simulink model "test_without_actuator"  (R2022b)
settings: Solver=FixedStepAuto  StartTime=0.0  StopTime=10  FixedStep=0.1  RelTol=1e-3
values from neighbouring files (symbols this model uses):
  C_M = 1.1366    [init.m]
  C_T = 3.5611    [init.m]
  D_p = 0.1    [init.m]
  model_param = struct(     'I', I,      'mass', ModelParam_m,      'g', ModelParam_g,      'c_T', ModelParam_c_T,      'c_M', ModelParam_c_M,      'd', ModelParam_d,      'J_RP', ModelParam_J_RP,      'init_pos', [ModelInit_Pos_x, ModelInit_Pos_y, ModelInit_Pos_z],      'init_att', [ModelInit_Att_x, ModelInit_Att_y, ModelInit_Att_z],      'C_T', C_T,      'C_M', C_M,      'air_density', p,      'prop_diameter',  ...(+52 chars)    [init.m]
  ModelInit_Att_qw = 0    [init.m]
  ModelInit_Att_qx = 1    [init.m]
  ModelInit_Att_qy = 0    [init.m]
  ModelInit_Att_qz = 0    [init.m]
  ModelInit_Pos_x = 0    [init.m]
  ModelInit_Pos_y = 0    [init.m]
  ModelInit_Pos_z = 0    [init.m]
  ModelParam_c_M = 1.779e-07*2    (= 3.558e-07)    [init.m]
  ModelParam_c_T = 1.105e-05    [init.m]
  ModelParam_d = 0.225    [init.m]
  ModelParam_g = 9.8    [init.m]
  ModelParam_I_xx = 0.0211    [init.m]
  ModelParam_I_yy = 0.0219    [init.m]
  ModelParam_I_zz = 0.0366    [init.m]
  ModelParam_J_RP = 0.0001287    [init.m]
  ModelParam_m = 1.4    [init.m]
  p = pos(idx,:)    [draw_morecool.m]    (also in init.m = 1.225)
(part 1 of 2)
settings Model: Creator=12854  LastModifiedBy=12854

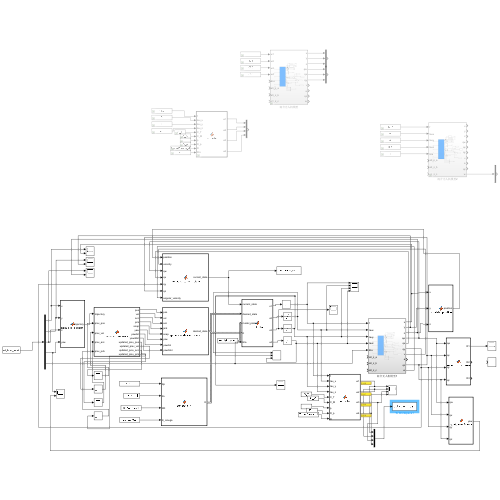
[thumbnail: Simulink's stored preview of the top-level diagram]
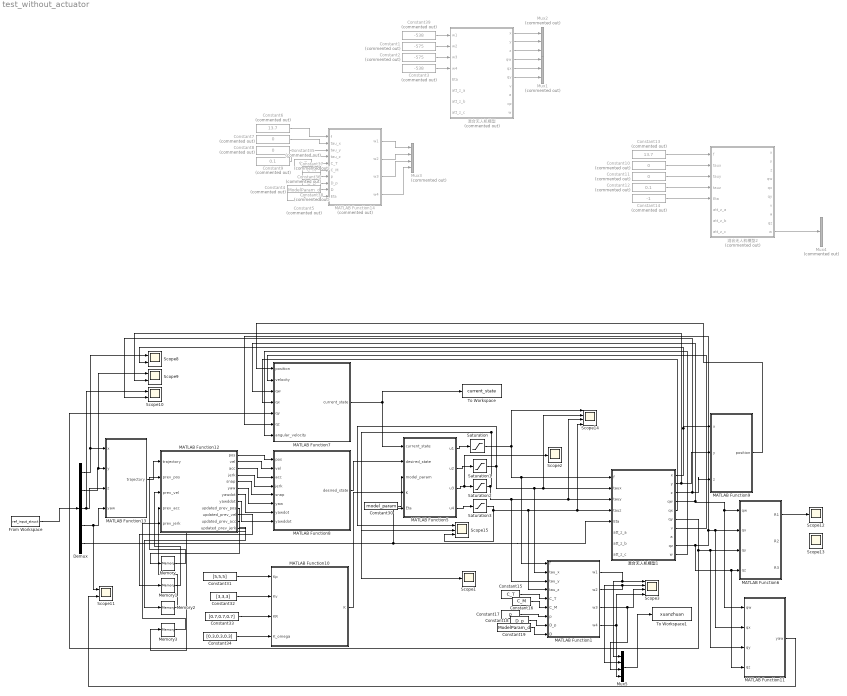
== system test_without_actuator ==
  Constant1 : Constant  Commented=on  Value=-575  SampleTime=0.1
  Constant10 : Constant  Commented=on  Value=0  SampleTime=0.1
  Constant11 : Constant  Commented=on  Value=0  SampleTime=0
  Constant12 : Constant  Commented=on  Value=0.1  SampleTime=0.1
  Constant13 : Constant  Commented=on  Value=13.7  SampleTime=0.1
  Constant14 : Constant  Commented=on  Value=-1  SampleTime=0.1
  Constant15 : Constant  Value=C_T  SampleTime=0.1
  Constant16 : Constant  Value=C_M  SampleTime=0.1
  Constant17 : Constant  Value=p  SampleTime=0.1
  Constant18 : Constant  Value=D_p  SampleTime=0.1
  Constant19 : Constant  Value=ModelParam_d  SampleTime=0.1
  Constant2 : Constant  Commented=on  Value=-575  SampleTime=0.1
  Constant3 : Constant  Commented=on  Value=-538  SampleTime=0.1
  Constant30 : Constant  Value=model_param  OutDataTypeStr=Bus: model_param_bus  SampleTime=0.1
  Constant31 : Constant  Value=[5,5,5]  SampleTime=0.1
  Constant32 : Constant  Value=[3,3,3]  SampleTime=0.1
  Constant33 : Constant  Value=[0.7,0.7,0.7]  SampleTime=0.1
  Constant34 : Constant  Value=[0.3,0.3,0.3]  SampleTime=0.1
  Constant35 : Constant  Commented=on  Value=C_T  SampleTime=0.1
  Constant36 : Constant  Commented=on  Value=C_M  SampleTime=0.1
  Constant37 : Constant  Commented=on  Value=p  SampleTime=0.1
  Constant38 : Constant  Commented=on  Value=D_p  SampleTime=0.1
  Constant39 : Constant  Commented=on  Value=-538  SampleTime=0.1
  Constant4 : Constant  Commented=on  Value=ModelParam_d  SampleTime=0.1
  Constant5 : Constant  Commented=on  Value=-1  SampleTime=0.1
  Constant6 : Constant  Commented=on  Value=13.7  SampleTime=0.1
  Constant7 : Constant  Commented=on  Value=0  SampleTime=0
  Constant8 : Constant  Commented=on  Value=0  SampleTime=0.1
  Constant9 : Constant  Commented=on  Value=0.1  SampleTime=0.1
  Demux : Demux  Outputs=5
  From Workspace : FromWorkspace  VariableName=ref_input_struct  SampleTime=0.1
  MATLAB Function1 : MATLAB Function  TreatAsAtomicUnit=on  SystemSampleTime=0.1
  MATLAB Function10 : MATLAB Function  TreatAsAtomicUnit=on
  MATLAB Function11 : MATLAB Function  TreatAsAtomicUnit=on
  MATLAB Function12 : MATLAB Function  TreatAsAtomicUnit=on
  MATLAB Function13 : MATLAB Function  TreatAsAtomicUnit=on
  MATLAB Function14 : MATLAB Function  Commented=on  TreatAsAtomicUnit=on  SystemSampleTime=0.1
  MATLAB Function5 : MATLAB Function  TreatAsAtomicUnit=on
  MATLAB Function6 : MATLAB Function  TreatAsAtomicUnit=on
  MATLAB Function7 : MATLAB Function  TreatAsAtomicUnit=on  SystemSampleTime=0.1
  MATLAB Function8 : MATLAB Function  TreatAsAtomicUnit=on
  MATLAB Function9 : MATLAB Function  TreatAsAtomicUnit=on
  Memory{,1..3} (4 alike) : Memory  InheritSampleTime=on
  Mux1 : Mux  Commented=on  Inputs=3
  Mux2 : Mux  Commented=on  Inputs=3
  Mux3 : Mux  Commented=on
  Mux4 : Mux  Commented=on  Inputs=1
  Mux5 : Mux
  Saturation : Saturate  UpperLimit=20  LowerLimit=-20
  Saturation1 : Saturate  UpperLimit=0.3  LowerLimit=-0.3
  Saturation2 : Saturate  UpperLimit=0.3  LowerLimit=-0.3
  Saturation3 : Saturate  UpperLimit=0.3  LowerLimit=-0.3
  Scope{1..2,12..13} (4 alike) : Scope
  Scope{8..11} (4 alike) : Scope  NumInputPorts=2
  Scope14 : Scope  NumInputPorts=4
  Scope15 : Scope  NumInputPorts=3
  Scope3 : Scope  NumInputPorts=4
  To Workspace : ToWorkspace  VariableName=current_state  SaveFormat=Timeseries  SampleTime=-1
  To Workspace1 : ToWorkspace  VariableName=xuanzhuan  SaveFormat=Timeseries  SampleTime=-1
  混合无人机模型 : Subsystem  Commented=on
  混合无人机模型1 : Subsystem
  混合无人机模型2 : Subsystem  Commented=on
  wires:
  Constant39/1 -> 混合无人机模型/1(w1)
  Constant1/1 -> 混合无人机模型/2(w2)
  Constant2/1 -> 混合无人机模型/3(w3)
  Constant3/1 -> 混合无人机模型/4(w4)
  混合无人机模型/1(x) -> Mux2/1
  混合无人机模型/2(y) -> Mux2/2
  混合无人机模型/3(z) -> Mux2/3
  混合无人机模型/4(qw) -> Mux1/1
  混合无人机模型/5(qx) -> Mux1/2
  混合无人机模型/6(qy) -> Mux1/3
  Constant35/1 -> MATLAB Function14/5(C_T)
  Constant36/1 -> MATLAB Function14/6(C_M)
  Constant37/1 -> MATLAB Function14/7(p)
  Constant38/1 -> MATLAB Function14/8(D_p)
  Constant4/1 -> MATLAB Function14/9(D)
  Constant5/1 -> MATLAB Function14/10(Eta)
  Constant6/1 -> MATLAB Function14/1(f)
  Constant7/1 -> MATLAB Function14/2(tau_x)
  Constant8/1 -> MATLAB Function14/3(tau_y)
  Constant9/1 -> MATLAB Function14/4(tau_z)
  MATLAB Function14/1(w1) -> Mux3/1
  MATLAB Function14/2(w2) -> Mux3/2
  MATLAB Function14/3(w3) -> Mux3/3
  MATLAB Function14/4(w4) -> Mux3/4
  MATLAB Function13/1(trajectory) -> MATLAB Function12/1(trajectory)
  MATLAB Function12/7(yawdot) -> MATLAB Function8/7(yawdot)
  MATLAB Function10/1(K) -> MATLAB Function5/4(K)
  MATLAB Function5/1(u1) -> Saturation/1
  Demux/1 -> Scope8/1, MATLAB Function13/1(x)
  Demux/2 -> Scope9/1, MATLAB Function13/2(y)
  混合无人机模型1/2(y) -> Scope9/2, MATLAB Function9/2(y)
  MATLAB Function5/4(u4) -> Saturation3/1
  From Workspace/1 -> Demux/1
  混合无人机模型1/7(v) -> MATLAB Function7/2(velocity)
  MATLAB Function6/1(R1) -> Scope12/1
  Constant31/1 -> MATLAB Function10/1(Kp)
  MATLAB Function12/10(updated_prev_vel) -> Memory1/1
  MATLAB Function7/1(current_state) -> MATLAB Function5/1(current_state), To Workspace/1
  混合无人机模型1/3(z) -> Scope10/2, MATLAB Function9/3(z)
  Memory1/1 -> MATLAB Function12/3(prev_vel)
  Constant32/1 -> MATLAB Function10/2(Kv)
  混合无人机模型1/10(w) -> MATLAB Function7/7(angular_velocity)
  Demux/4 -> Scope11/1, MATLAB Function13/4(yaw)
  MATLAB Function12/6(yaw) -> MATLAB Function8/6(yaw)
  Memory3/1 -> MATLAB Function12/5(prev_jerk)
  Constant34/1 -> MATLAB Function10/4(K_omega)
  MATLAB Function12/1(pos) -> MATLAB Function8/1(pos)
  Memory/1 -> MATLAB Function12/2(prev_pos)
  MATLAB Function12/5(snap) -> MATLAB Function8/5(snap)
  MATLAB Function8/1(desired_state) -> MATLAB Function5/2(desired_state)
  MATLAB Function9/1(position) -> MATLAB Function7/1(position)
  Constant33/1 -> MATLAB Function10/3(KR)
  MATLAB Function12/4(jerk) -> MATLAB Function8/4(jerk)
  MATLAB Function5/2(u2) -> Saturation1/1
  混合无人机模型1/1(x) -> Scope8/2, MATLAB Function9/1(x)
  Constant30/1 -> MATLAB Function5/3(model_param)
  MATLAB Function12/11(updated_prev_acc) -> Memory2/1
  混合无人机模型1/5(qx) -> MATLAB Function7/4(qx)
  MATLAB Function12/2(vel) -> MATLAB Function8/2(vel)
  混合无人机模型1/4(qw) -> MATLAB Function7/3(qw), MATLAB Function11/1(qw), MATLAB Function6/1(qw)
  Demux/3 -> Scope10/1, MATLAB Function13/3(z)
  MATLAB Function12/3(acc) -> MATLAB Function8/3(acc)
  混合无人机模型1/6(qy) -> MATLAB Function11/3(qy), MATLAB Function6/3(qy), MATLAB Function7/5(qy)
  Demux/5 -> MATLAB Function5/5(Eta), 混合无人机模型1/5(Eta)
  MATLAB Function11/1(yaw) -> Scope11/2
  MATLAB Function12/9(updated_prev_pos) -> Memory/1
  MATLAB Function12/12(updated_prev_jerk) -> Memory3/1
  Memory2/1 -> MATLAB Function12/4(prev_acc)
  Saturation3/1 -> MATLAB Function1/4(tau_z), Scope14/4, 混合无人机模型1/4(tauz), Scope15/3
  混合无人机模型1/9(qz) -> MATLAB Function11/4(qz), MATLAB Function6/4(qz), MATLAB Function7/6(qz), MATLAB Function11/2(qx), MATLAB Function6/2(qx)
  MATLAB Function5/3(u3) -> Scope2/1, Saturation2/1
  MATLAB Function12/8(yawddot) -> MATLAB Function8/8(yawddot)
  Constant13/1 -> 混合无人机模型2/1(f)
  Constant10/1 -> 混合无人机模型2/2(taux)
  Constant11/1 -> 混合无人机模型2/3(tauy)
  Constant12/1 -> 混合无人机模型2/4(tauz)
  Constant14/1 -> 混合无人机模型2/5(Eta)
  混合无人机模型2/10(w) -> Mux4/1
  Saturation/1 -> Scope14/1, MATLAB Function1/1(f), 混合无人机模型1/1(f)
  Saturation2/1 -> MATLAB Function1/3(tau_y), Scope14/3, 混合无人机模型1/3(tauy), Scope15/2, Scope1/1
  Constant15/1 -> MATLAB Function1/5(C_T)
  Constant17/1 -> MATLAB Function1/7(p)
  Constant16/1 -> MATLAB Function1/6(C_M)
  Constant18/1 -> MATLAB Function1/8(D_p)
  Constant19/1 -> MATLAB Function1/9(D)
  Saturation1/1 -> Scope15/1, MATLAB Function1/2(tau_x), Scope14/2, 混合无人机模型1/2(taux)
  MATLAB Function1/1(w1) -> Scope3/1, Mux5/1
  MATLAB Function1/2(w2) -> Scope3/2, Mux5/2
  MATLAB Function1/4(w4) -> Mux5/4, Scope3/4
  Mux5/1 -> To Workspace1/1
  MATLAB Function1/3(w3) -> Mux5/3, Scope3/3

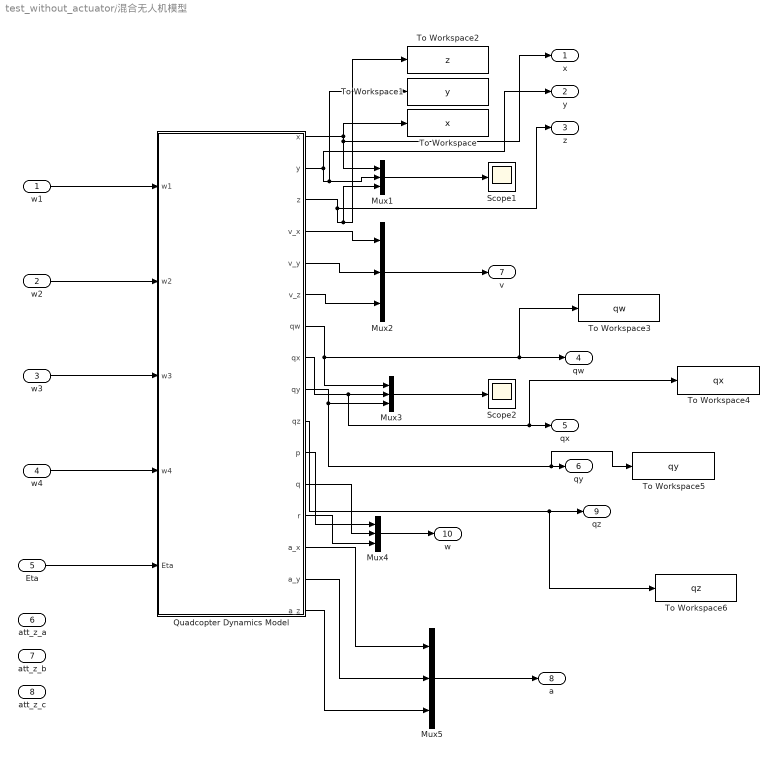
== system test_without_actuator/混合无人机模型 ==
  w1 : Inport
  w2 : Inport  Port=2
  w3 : Inport  Port=3
  w4 : Inport  Port=4
  Eta : Inport  Port=5
  att_z_a : Inport  Port=6
  att_z_b : Inport  Port=7
  att_z_c : Inport  Port=8
  Mux{1..5} (5 alike) : Mux  Inputs=3
  Quadcopter Dynamics Model : Subsystem
  Scope1 : Scope
  Scope2 : Scope
  To Workspace : ToWorkspace  VariableName=x  SaveFormat=Timeseries  SampleTime=-1
  To Workspace1 : ToWorkspace  VariableName=y  SaveFormat=Timeseries  SampleTime=-1
  To Workspace2 : ToWorkspace  VariableName=z  SaveFormat=Timeseries  SampleTime=-1
  To Workspace3 : ToWorkspace  VariableName=qw  SaveFormat=Timeseries  SampleTime=-1
  To Workspace4 : ToWorkspace  VariableName=qx  SaveFormat=Timeseries  SampleTime=-1
  To Workspace5 : ToWorkspace  VariableName=qy  SaveFormat=Timeseries  SampleTime=-1
  To Workspace6 : ToWorkspace  VariableName=qz  SaveFormat=Timeseries  SampleTime=-1
  x : Outport
  y : Outport  Port=2
  z : Outport  Port=3
  qw : Outport  Port=4
  qx : Outport  Port=5
  qy : Outport  Port=6
  v : Outport  Port=7
  a : Outport  Port=8
  qz : Outport  Port=9
  w : Outport  Port=10
  wires:
  Mux3/1 -> Scope2/1
  Quadcopter Dynamics Model/2(y) -> To Workspace1/1, Mux1/2, y/1
  Quadcopter Dynamics Model/8(qx) -> To Workspace4/1, qx/1, Mux3/2
  Quadcopter Dynamics Model/5(v_y) -> Mux2/2
  Quadcopter Dynamics Model/1(x) -> Mux1/1, x/1, To Workspace/1
  Quadcopter Dynamics Model/6(v_z) -> Mux2/3
  Mux2/1 -> v/1
  Quadcopter Dynamics Model/13(r) -> Mux4/3
  Mux1/1 -> Scope1/1
  Quadcopter Dynamics Model/11(p) -> Mux4/1
  Quadcopter Dynamics Model/4(v_x) -> Mux2/1
  Quadcopter Dynamics Model/7(qw) -> Mux3/1, To Workspace3/1, qw/1
  Quadcopter Dynamics Model/3(z) -> To Workspace2/1, Mux1/3, z/1
  Quadcopter Dynamics Model/12(q) -> Mux4/2
  Quadcopter Dynamics Model/9(qy) -> To Workspace5/1, qy/1, Mux3/3
  w1/1 -> Quadcopter Dynamics Model/1(w1)
  w2/1 -> Quadcopter Dynamics Model/2(w2)
  w3/1 -> Quadcopter Dynamics Model/3(w3)
  w4/1 -> Quadcopter Dynamics Model/4(w4)
  Quadcopter Dynamics Model/16(a_z) -> Mux5/3
  Quadcopter Dynamics Model/15(a_y) -> Mux5/2
  Quadcopter Dynamics Model/14(a_x) -> Mux5/1
  Mux5/1 -> a/1
  Quadcopter Dynamics Model/10(qz) -> To Workspace6/1, qz/1
  Eta/1 -> Quadcopter Dynamics Model/5(Eta)
  Mux4/1 -> w/1

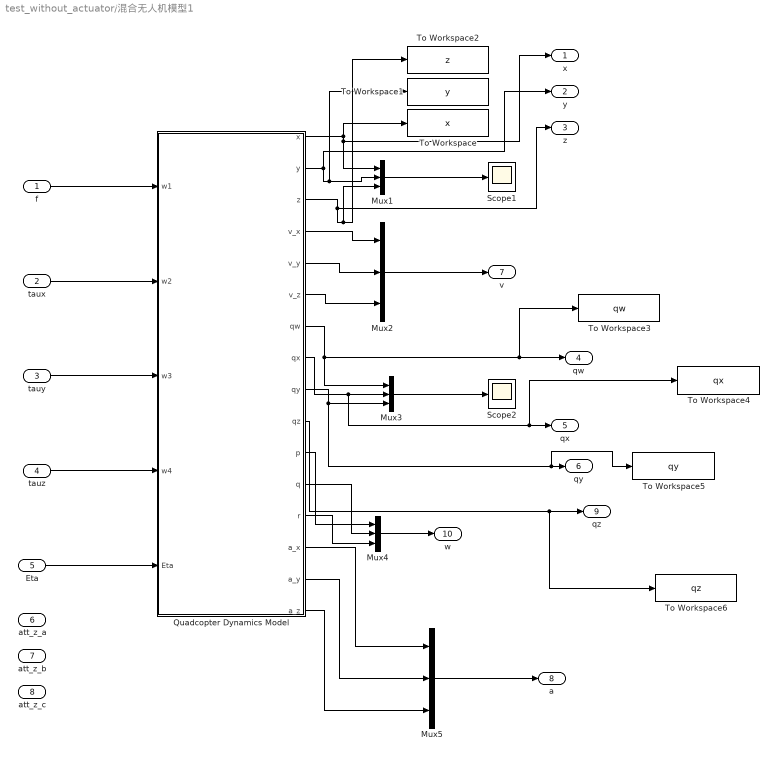
== system test_without_actuator/混合无人机模型1 ==
  f : Inport  SampleTime=0.1
  taux : Inport  Port=2  SampleTime=0.1
  tauy : Inport  Port=3  SampleTime=0.1
  tauz : Inport  Port=4  SampleTime=0.1
  Eta : Inport  Port=5  SampleTime=0.1
  att_z_a : Inport  Port=6
  att_z_b : Inport  Port=7
  att_z_c : Inport  Port=8
  Mux{1..5} (5 alike) : Mux  Inputs=3
  Quadcopter Dynamics Model : Subsystem
  Scope1 : Scope
  Scope2 : Scope
  To Workspace : ToWorkspace  VariableName=x  SaveFormat=Timeseries  SampleTime=-1
  To Workspace1 : ToWorkspace  VariableName=y  SaveFormat=Timeseries  SampleTime=-1
  To Workspace2 : ToWorkspace  VariableName=z  SaveFormat=Timeseries  SampleTime=-1
  To Workspace3 : ToWorkspace  VariableName=qw  SaveFormat=Timeseries  SampleTime=-1
  To Workspace4 : ToWorkspace  VariableName=qx  SaveFormat=Timeseries  SampleTime=-1
  To Workspace5 : ToWorkspace  VariableName=qy  SaveFormat=Timeseries  SampleTime=-1
  To Workspace6 : ToWorkspace  VariableName=qz  SaveFormat=Timeseries  SampleTime=-1
  x : Outport
  y : Outport  Port=2
  z : Outport  Port=3
  qw : Outport  Port=4
  qx : Outport  Port=5
  qy : Outport  Port=6
  v : Outport  Port=7
  a : Outport  Port=8
  qz : Outport  Port=9
  w : Outport  Port=10
  wires:
  Mux3/1 -> Scope2/1
  Quadcopter Dynamics Model/2(y) -> To Workspace1/1, Mux1/2, y/1
  Quadcopter Dynamics Model/8(qx) -> To Workspace4/1, qx/1, Mux3/2
  Quadcopter Dynamics Model/5(v_y) -> Mux2/2
  Quadcopter Dynamics Model/1(x) -> Mux1/1, x/1, To Workspace/1
  Quadcopter Dynamics Model/6(v_z) -> Mux2/3
  Mux2/1 -> v/1
  Quadcopter Dynamics Model/13(r) -> Mux4/3
  Mux1/1 -> Scope1/1
  Quadcopter Dynamics Model/11(p) -> Mux4/1
  Quadcopter Dynamics Model/4(v_x) -> Mux2/1
  Quadcopter Dynamics Model/7(qw) -> Mux3/1, To Workspace3/1, qw/1
  Quadcopter Dynamics Model/3(z) -> To Workspace2/1, Mux1/3, z/1
  Quadcopter Dynamics Model/12(q) -> Mux4/2
  Quadcopter Dynamics Model/9(qy) -> To Workspace5/1, qy/1, Mux3/3
  f/1 -> Quadcopter Dynamics Model/1(w1)
  taux/1 -> Quadcopter Dynamics Model/2(w2)
  tauy/1 -> Quadcopter Dynamics Model/3(w3)
  tauz/1 -> Quadcopter Dynamics Model/4(w4)
  Quadcopter Dynamics Model/16(a_z) -> Mux5/3
  Quadcopter Dynamics Model/15(a_y) -> Mux5/2
  Quadcopter Dynamics Model/14(a_x) -> Mux5/1
  Mux5/1 -> a/1
  Quadcopter Dynamics Model/10(qz) -> To Workspace6/1, qz/1
  Eta/1 -> Quadcopter Dynamics Model/5(Eta)
  Mux4/1 -> w/1

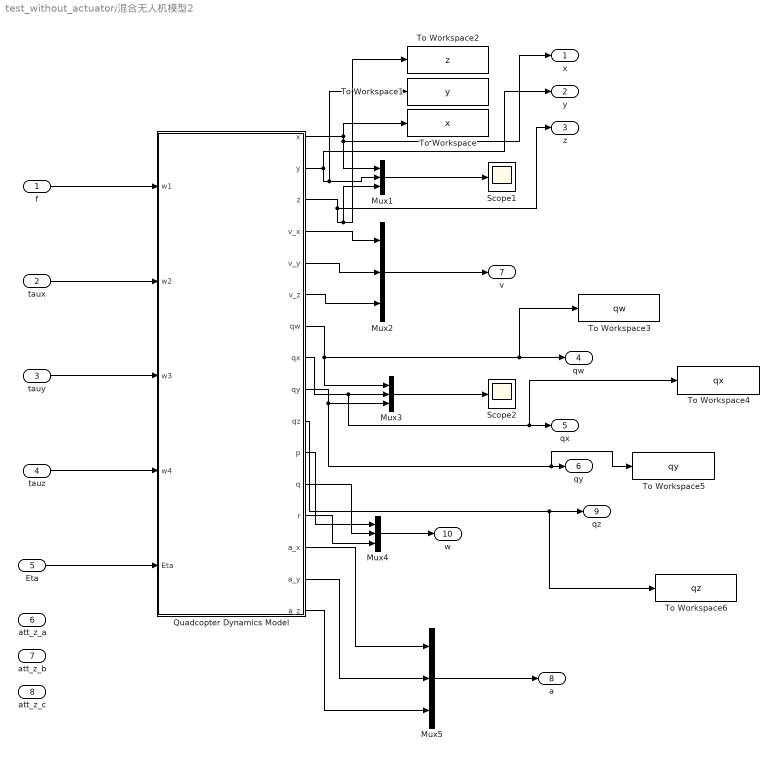
== system test_without_actuator/混合无人机模型2 ==
  f : Inport  SampleTime=0.1
  taux : Inport  Port=2  SampleTime=0.1
  tauy : Inport  Port=3  SampleTime=0.1
  tauz : Inport  Port=4  SampleTime=0.1
  Eta : Inport  Port=5  SampleTime=0.1
  att_z_a : Inport  Port=6
  att_z_b : Inport  Port=7
  att_z_c : Inport  Port=8
  Mux{1..5} (5 alike) : Mux  Inputs=3
  Quadcopter Dynamics Model : Subsystem
  Scope1 : Scope
  Scope2 : Scope
  To Workspace : ToWorkspace  VariableName=x  SaveFormat=Timeseries  SampleTime=-1
  To Workspace1 : ToWorkspace  VariableName=y  SaveFormat=Timeseries  SampleTime=-1
  To Workspace2 : ToWorkspace  VariableName=z  SaveFormat=Timeseries  SampleTime=-1
  To Workspace3 : ToWorkspace  VariableName=qw  SaveFormat=Timeseries  SampleTime=-1
  To Workspace4 : ToWorkspace  VariableName=qx  SaveFormat=Timeseries  SampleTime=-1
  To Workspace5 : ToWorkspace  VariableName=qy  SaveFormat=Timeseries  SampleTime=-1
  To Workspace6 : ToWorkspace  VariableName=qz  SaveFormat=Timeseries  SampleTime=-1
  x : Outport
  y : Outport  Port=2
  z : Outport  Port=3
  qw : Outport  Port=4
  qx : Outport  Port=5
  qy : Outport  Port=6
  v : Outport  Port=7
  a : Outport  Port=8
  qz : Outport  Port=9
  w : Outport  Port=10
  wires:
  Mux3/1 -> Scope2/1
  Quadcopter Dynamics Model/2(y) -> To Workspace1/1, Mux1/2, y/1
  Quadcopter Dynamics Model/8(qx) -> To Workspace4/1, qx/1, Mux3/2
  Quadcopter Dynamics Model/5(v_y) -> Mux2/2
  Quadcopter Dynamics Model/1(x) -> Mux1/1, x/1, To Workspace/1
  Quadcopter Dynamics Model/6(v_z) -> Mux2/3
  Mux2/1 -> v/1
  Quadcopter Dynamics Model/13(r) -> Mux4/3
  Mux1/1 -> Scope1/1
  Quadcopter Dynamics Model/11(p) -> Mux4/1
  Quadcopter Dynamics Model/4(v_x) -> Mux2/1
  Quadcopter Dynamics Model/7(qw) -> Mux3/1, To Workspace3/1, qw/1
  Quadcopter Dynamics Model/3(z) -> To Workspace2/1, Mux1/3, z/1
  Quadcopter Dynamics Model/12(q) -> Mux4/2
  Quadcopter Dynamics Model/9(qy) -> To Workspace5/1, qy/1, Mux3/3
  f/1 -> Quadcopter Dynamics Model/1(w1)
  taux/1 -> Quadcopter Dynamics Model/2(w2)
  tauy/1 -> Quadcopter Dynamics Model/3(w3)
  tauz/1 -> Quadcopter Dynamics Model/4(w4)
  Quadcopter Dynamics Model/16(a_z) -> Mux5/3
  Quadcopter Dynamics Model/15(a_y) -> Mux5/2
  Quadcopter Dynamics Model/14(a_x) -> Mux5/1
  Mux5/1 -> a/1
  Quadcopter Dynamics Model/10(qz) -> To Workspace6/1, qz/1
  Eta/1 -> Quadcopter Dynamics Model/5(Eta)
  Mux4/1 -> w/1

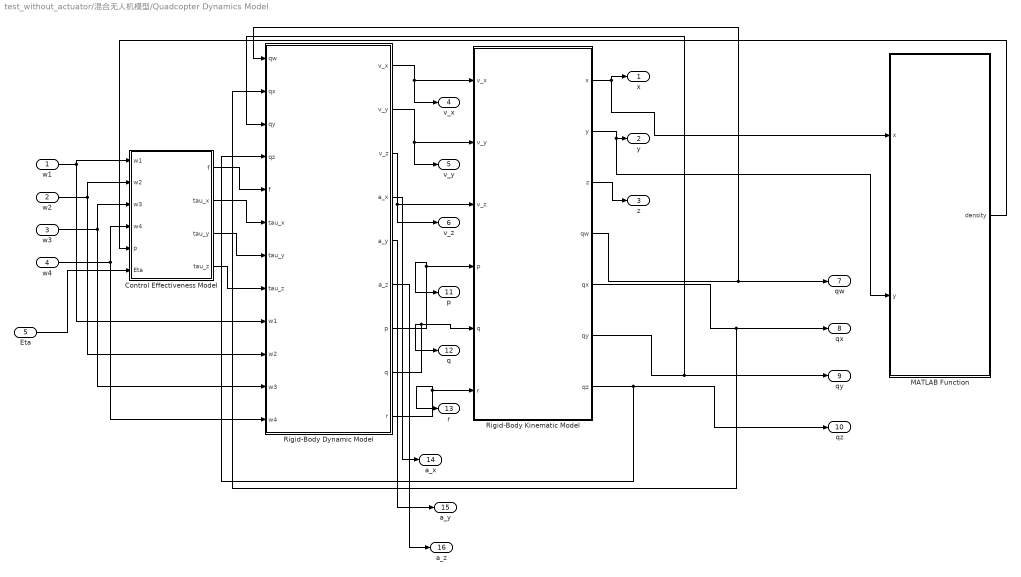
== system test_without_actuator/混合无人机模型/Quadcopter Dynamics Model ==
  w1 : Inport
  w2 : Inport  Port=2
  w3 : Inport  Port=3
  w4 : Inport  Port=4
  Eta : Inport  Port=5
  Control Effectiveness Model : Subsystem
  MATLAB Function : MATLAB Function  TreatAsAtomicUnit=on
  Rigid-Body Dynamic Model : Subsystem
  Rigid-Body Kinematic Model : Subsystem
  x : Outport  VectorParamsAs1DForOutWhenUnconnected=off
  y : Outport  Port=2  VectorParamsAs1DForOutWhenUnconnected=off
  z : Outport  Port=3  VectorParamsAs1DForOutWhenUnconnected=off
  v_x : Outport  Port=4  VectorParamsAs1DForOutWhenUnconnected=off
  v_y : Outport  Port=5  VectorParamsAs1DForOutWhenUnconnected=off
  v_z : Outport  Port=6  VectorParamsAs1DForOutWhenUnconnected=off
  qw : Outport  Port=7  VectorParamsAs1DForOutWhenUnconnected=off
  qx : Outport  Port=8  VectorParamsAs1DForOutWhenUnconnected=off
  qy : Outport  Port=9  VectorParamsAs1DForOutWhenUnconnected=off
  qz : Outport  Port=10  VectorParamsAs1DForOutWhenUnconnected=off
  p : Outport  Port=11  VectorParamsAs1DForOutWhenUnconnected=off
  q : Outport  Port=12  VectorParamsAs1DForOutWhenUnconnected=off
  r : Outport  Port=13  VectorParamsAs1DForOutWhenUnconnected=off
  a_x : Outport  Port=14  VectorParamsAs1DForOutWhenUnconnected=off
  a_y : Outport  Port=15  VectorParamsAs1DForOutWhenUnconnected=off
  a_z : Outport  Port=16  VectorParamsAs1DForOutWhenUnconnected=off
  wires:
  w1/1 -> Rigid-Body Dynamic Model/9(w1), Control Effectiveness Model/1(w1)
  w3/1 -> Rigid-Body Dynamic Model/11(w3), Control Effectiveness Model/3(w3)
  w4/1 -> Rigid-Body Dynamic Model/12(w4), Control Effectiveness Model/4(w4)
  w2/1 -> Control Effectiveness Model/2(w2), Rigid-Body Dynamic Model/10(w2)
  Rigid-Body Dynamic Model/7(p) -> p/1, Rigid-Body Kinematic Model/4(p)
  Rigid-Body Dynamic Model/9(r) -> r/1, Rigid-Body Kinematic Model/6(r)
  Control Effectiveness Model/2(tau_x) -> Rigid-Body Dynamic Model/6(tau_x)
  Rigid-Body Kinematic Model/1(x) -> x/1, MATLAB Function/1(x)
  Rigid-Body Dynamic Model/8(q) -> q/1, Rigid-Body Kinematic Model/5(q)
  Control Effectiveness Model/4(tau_z) -> Rigid-Body Dynamic Model/8(tau_z)
  Rigid-Body Kinematic Model/2(y) -> MATLAB Function/2(y), y/1
  Rigid-Body Kinematic Model/3(z) -> z/1
  Control Effectiveness Model/3(tau_y) -> Rigid-Body Dynamic Model/7(tau_y)
  Rigid-Body Kinematic Model/4(qw) -> Rigid-Body Dynamic Model/1(qw), qw/1
  Rigid-Body Kinematic Model/5(qx) -> Rigid-Body Dynamic Model/2(qx), qx/1
  Rigid-Body Kinematic Model/6(qy) -> Rigid-Body Dynamic Model/3(qy), qy/1
  MATLAB Function/1(density) -> Control Effectiveness Model/5(p)
  Rigid-Body Dynamic Model/4(a_x) -> a_x/1
  Rigid-Body Dynamic Model/5(a_y) -> a_y/1
  Rigid-Body Dynamic Model/6(a_z) -> a_z/1
  Rigid-Body Dynamic Model/1(v_x) -> Rigid-Body Kinematic Model/1(v_x), v_x/1
  Rigid-Body Dynamic Model/2(v_y) -> Rigid-Body Kinematic Model/2(v_y), v_y/1
  Rigid-Body Dynamic Model/3(v_z) -> Rigid-Body Kinematic Model/3(v_z), v_z/1
  Control Effectiveness Model/1(f) -> Rigid-Body Dynamic Model/5(f)
  Rigid-Body Kinematic Model/7(qz) -> Rigid-Body Dynamic Model/4(qz), qz/1
  Eta/1 -> Control Effectiveness Model/6(Eta)

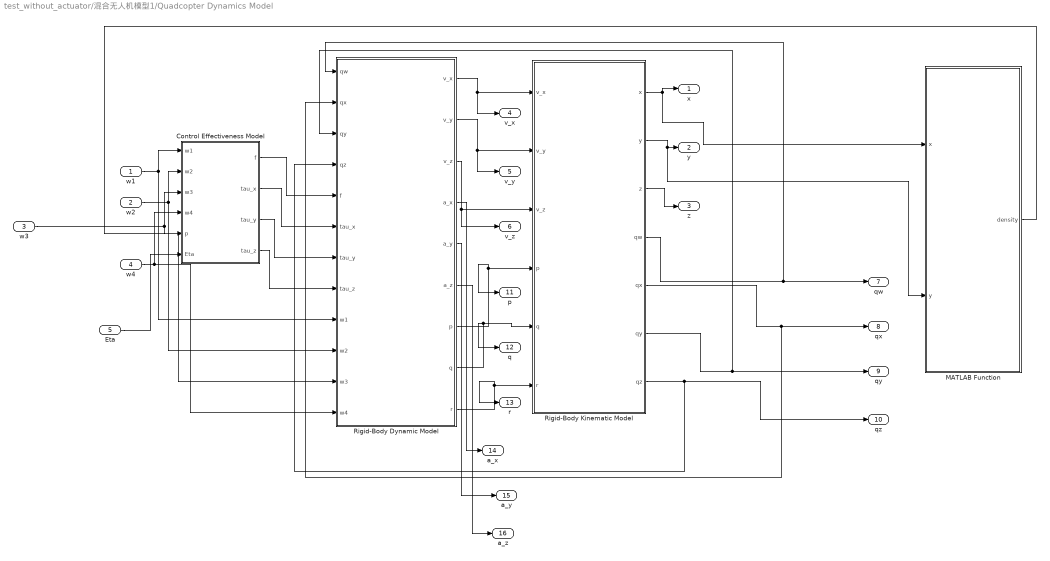
== system test_without_actuator/混合无人机模型1/Quadcopter Dynamics Model ==
  w1 : Inport  SampleTime=0.1
  w2 : Inport  Port=2  SampleTime=0.1
  w3 : Inport  Port=3  SampleTime=0.1
  w4 : Inport  Port=4
  Eta : Inport  Port=5  SampleTime=0.1
  Control Effectiveness Model : Subsystem
  MATLAB Function : MATLAB Function  TreatAsAtomicUnit=on
  Rigid-Body Dynamic Model : Subsystem
  Rigid-Body Kinematic Model : Subsystem
  x : Outport  VectorParamsAs1DForOutWhenUnconnected=off
  y : Outport  Port=2  VectorParamsAs1DForOutWhenUnconnected=off
  z : Outport  Port=3  VectorParamsAs1DForOutWhenUnconnected=off
  v_x : Outport  Port=4  VectorParamsAs1DForOutWhenUnconnected=off
  v_y : Outport  Port=5  VectorParamsAs1DForOutWhenUnconnected=off
  v_z : Outport  Port=6  VectorParamsAs1DForOutWhenUnconnected=off
  qw : Outport  Port=7  VectorParamsAs1DForOutWhenUnconnected=off
  qx : Outport  Port=8  VectorParamsAs1DForOutWhenUnconnected=off
  qy : Outport  Port=9  VectorParamsAs1DForOutWhenUnconnected=off
  qz : Outport  Port=10  VectorParamsAs1DForOutWhenUnconnected=off
  p : Outport  Port=11  VectorParamsAs1DForOutWhenUnconnected=off
  q : Outport  Port=12  VectorParamsAs1DForOutWhenUnconnected=off
  r : Outport  Port=13  VectorParamsAs1DForOutWhenUnconnected=off
  a_x : Outport  Port=14  VectorParamsAs1DForOutWhenUnconnected=off
  a_y : Outport  Port=15  VectorParamsAs1DForOutWhenUnconnected=off
  a_z : Outport  Port=16  VectorParamsAs1DForOutWhenUnconnected=off
  wires:
  w1/1 -> Rigid-Body Dynamic Model/9(w1), Control Effectiveness Model/1(w1)
  w3/1 -> Rigid-Body Dynamic Model/11(w3), Control Effectiveness Model/3(w3)
  w4/1 -> Rigid-Body Dynamic Model/12(w4), Control Effectiveness Model/4(w4)
  w2/1 -> Control Effectiveness Model/2(w2), Rigid-Body Dynamic Model/10(w2)
  Rigid-Body Dynamic Model/7(p) -> p/1, Rigid-Body Kinematic Model/4(p)
  Rigid-Body Dynamic Model/9(r) -> r/1, Rigid-Body Kinematic Model/6(r)
  Control Effectiveness Model/2(tau_x) -> Rigid-Body Dynamic Model/6(tau_x)
  Rigid-Body Kinematic Model/1(x) -> x/1, MATLAB Function/1(x)
  Rigid-Body Dynamic Model/8(q) -> q/1, Rigid-Body Kinematic Model/5(q)
  Control Effectiveness Model/4(tau_z) -> Rigid-Body Dynamic Model/8(tau_z)
  Rigid-Body Kinematic Model/2(y) -> MATLAB Function/2(y), y/1
  Rigid-Body Kinematic Model/3(z) -> z/1
  Control Effectiveness Model/3(tau_y) -> Rigid-Body Dynamic Model/7(tau_y)
  Rigid-Body Kinematic Model/4(qw) -> Rigid-Body Dynamic Model/1(qw), qw/1
  Rigid-Body Kinematic Model/5(qx) -> Rigid-Body Dynamic Model/2(qx), qx/1
  Rigid-Body Kinematic Model/6(qy) -> Rigid-Body Dynamic Model/3(qy), qy/1
  MATLAB Function/1(density) -> Control Effectiveness Model/5(p)
  Rigid-Body Dynamic Model/4(a_x) -> a_x/1
  Rigid-Body Dynamic Model/5(a_y) -> a_y/1
  Rigid-Body Dynamic Model/6(a_z) -> a_z/1
  Rigid-Body Dynamic Model/1(v_x) -> Rigid-Body Kinematic Model/1(v_x), v_x/1
  Rigid-Body Dynamic Model/2(v_y) -> Rigid-Body Kinematic Model/2(v_y), v_y/1
  Rigid-Body Dynamic Model/3(v_z) -> Rigid-Body Kinematic Model/3(v_z), v_z/1
  Control Effectiveness Model/1(f) -> Rigid-Body Dynamic Model/5(f)
  Rigid-Body Kinematic Model/7(qz) -> Rigid-Body Dynamic Model/4(qz), qz/1
  Eta/1 -> Control Effectiveness Model/6(Eta)

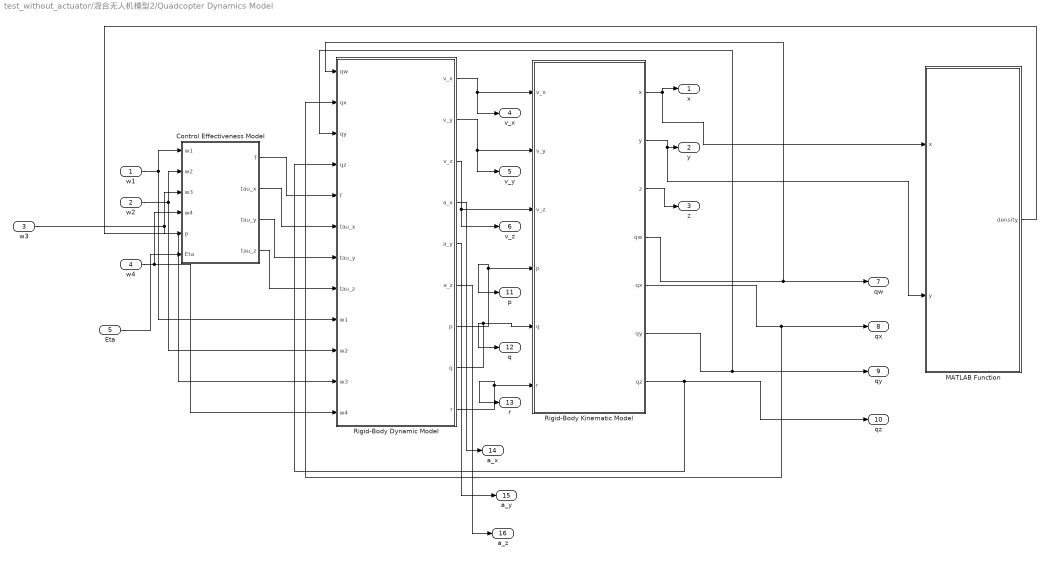
== system test_without_actuator/混合无人机模型2/Quadcopter Dynamics Model ==
  w1 : Inport  SampleTime=0.1
  w2 : Inport  Port=2  SampleTime=0.1
  w3 : Inport  Port=3  SampleTime=0.1
  w4 : Inport  Port=4
  Eta : Inport  Port=5  SampleTime=0.1
  Control Effectiveness Model : Subsystem
  MATLAB Function : MATLAB Function  TreatAsAtomicUnit=on
  Rigid-Body Dynamic Model : Subsystem
  Rigid-Body Kinematic Model : Subsystem
  x : Outport  VectorParamsAs1DForOutWhenUnconnected=off
  y : Outport  Port=2  VectorParamsAs1DForOutWhenUnconnected=off
  z : Outport  Port=3  VectorParamsAs1DForOutWhenUnconnected=off
  v_x : Outport  Port=4  VectorParamsAs1DForOutWhenUnconnected=off
  v_y : Outport  Port=5  VectorParamsAs1DForOutWhenUnconnected=off
  v_z : Outport  Port=6  VectorParamsAs1DForOutWhenUnconnected=off
  qw : Outport  Port=7  VectorParamsAs1DForOutWhenUnconnected=off
  qx : Outport  Port=8  VectorParamsAs1DForOutWhenUnconnected=off
  qy : Outport  Port=9  VectorParamsAs1DForOutWhenUnconnected=off
  qz : Outport  Port=10  VectorParamsAs1DForOutWhenUnconnected=off
  p : Outport  Port=11  VectorParamsAs1DForOutWhenUnconnected=off
  q : Outport  Port=12  VectorParamsAs1DForOutWhenUnconnected=off
  r : Outport  Port=13  VectorParamsAs1DForOutWhenUnconnected=off
  a_x : Outport  Port=14  VectorParamsAs1DForOutWhenUnconnected=off
  a_y : Outport  Port=15  VectorParamsAs1DForOutWhenUnconnected=off
  a_z : Outport  Port=16  VectorParamsAs1DForOutWhenUnconnected=off
  wires:
  w1/1 -> Rigid-Body Dynamic Model/9(w1), Control Effectiveness Model/1(w1)
  w3/1 -> Rigid-Body Dynamic Model/11(w3), Control Effectiveness Model/3(w3)
  w4/1 -> Rigid-Body Dynamic Model/12(w4), Control Effectiveness Model/4(w4)
  w2/1 -> Control Effectiveness Model/2(w2), Rigid-Body Dynamic Model/10(w2)
  Rigid-Body Dynamic Model/7(p) -> p/1, Rigid-Body Kinematic Model/4(p)
  Rigid-Body Dynamic Model/9(r) -> r/1, Rigid-Body Kinematic Model/6(r)
  Control Effectiveness Model/2(tau_x) -> Rigid-Body Dynamic Model/6(tau_x)
  Rigid-Body Kinematic Model/1(x) -> x/1, MATLAB Function/1(x)
  Rigid-Body Dynamic Model/8(q) -> q/1, Rigid-Body Kinematic Model/5(q)
  Control Effectiveness Model/4(tau_z) -> Rigid-Body Dynamic Model/8(tau_z)
  Rigid-Body Kinematic Model/2(y) -> MATLAB Function/2(y), y/1
  Rigid-Body Kinematic Model/3(z) -> z/1
  Control Effectiveness Model/3(tau_y) -> Rigid-Body Dynamic Model/7(tau_y)
  Rigid-Body Kinematic Model/4(qw) -> Rigid-Body Dynamic Model/1(qw), qw/1
  Rigid-Body Kinematic Model/5(qx) -> Rigid-Body Dynamic Model/2(qx), qx/1
  Rigid-Body Kinematic Model/6(qy) -> Rigid-Body Dynamic Model/3(qy), qy/1
  MATLAB Function/1(density) -> Control Effectiveness Model/5(p)
  Rigid-Body Dynamic Model/4(a_x) -> a_x/1
  Rigid-Body Dynamic Model/5(a_y) -> a_y/1
  Rigid-Body Dynamic Model/6(a_z) -> a_z/1
  Rigid-Body Dynamic Model/1(v_x) -> Rigid-Body Kinematic Model/1(v_x), v_x/1
  Rigid-Body Dynamic Model/2(v_y) -> Rigid-Body Kinematic Model/2(v_y), v_y/1
  Rigid-Body Dynamic Model/3(v_z) -> Rigid-Body Kinematic Model/3(v_z), v_z/1
  Control Effectiveness Model/1(f) -> Rigid-Body Dynamic Model/5(f)
  Rigid-Body Kinematic Model/7(qz) -> Rigid-Body Dynamic Model/4(qz), qz/1
  Eta/1 -> Control Effectiveness Model/6(Eta)

== system test_without_actuator/混合无人机模型/Quadcopter Dynamics Model/Control Effectiveness Model ==
  w1 : Inport
  w2 : Inport  Port=2
  w3 : Inport  Port=3
  w4 : Inport  Port=4
  p : Inport  Port=5
  Eta : Inport  Port=6
  Constant : Constant  Value=ModelParam_c_T
  Constant1 : Constant  Value=ModelParam_c_M
  Constant2 : Constant  Value=ModelParam_d
  MATLAB Function : MATLAB Function  TreatAsAtomicUnit=on  SystemSampleTime=0.1
  f : Outport  VectorParamsAs1DForOutWhenUnconnected=off
  tau_x : Outport  Port=2  VectorParamsAs1DForOutWhenUnconnected=off
  tau_y : Outport  Port=3  VectorParamsAs1DForOutWhenUnconnected=off
  tau_z : Outport  Port=4  VectorParamsAs1DForOutWhenUnconnected=off
  wires:
  Constant1/1 -> MATLAB Function/6(c_M)
  Constant/1 -> MATLAB Function/5(c_T)
  MATLAB Function/3(tau_y) -> tau_y/1
  MATLAB Function/1(f) -> f/1
  Constant2/1 -> MATLAB Function/7(d)
  MATLAB Function/4(tau_z) -> tau_z/1
  w3/1 -> MATLAB Function/3(w3)
  w1/1 -> MATLAB Function/1(w1)
  w4/1 -> MATLAB Function/4(w4)
  MATLAB Function/2(tau_x) -> tau_x/1
  w2/1 -> MATLAB Function/2(w2)
  p/1 -> MATLAB Function/8(p)
  Eta/1 -> MATLAB Function/9(Eta)

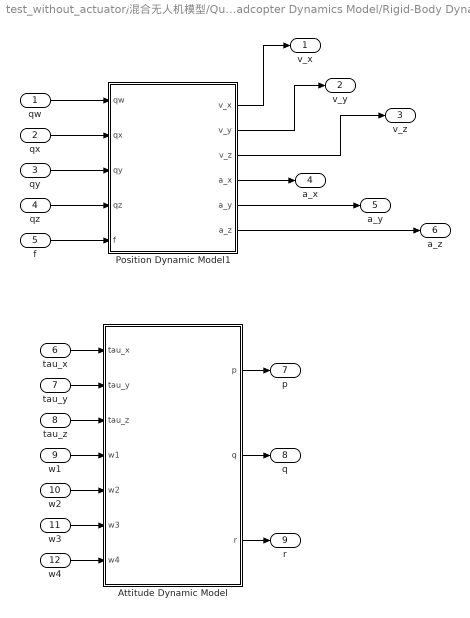
== system test_without_actuator/混合无人机模型/Quadcopter Dynamics Model/Rigid-Body Dynamic Model ==
  qw : Inport
  qx : Inport  Port=2
  qy : Inport  Port=3
  qz : Inport  Port=4
  f : Inport  Port=5
  tau_x : Inport  Port=6
  tau_y : Inport  Port=7
  tau_z : Inport  Port=8
  w1 : Inport  Port=9
  w2 : Inport  Port=10
  w3 : Inport  Port=11
  w4 : Inport  Port=12
  Attitude Dynamic Model : Subsystem
  Position Dynamic Model1 : Subsystem
  v_x : Outport  VectorParamsAs1DForOutWhenUnconnected=off
  v_y : Outport  Port=2  VectorParamsAs1DForOutWhenUnconnected=off
  v_z : Outport  Port=3  VectorParamsAs1DForOutWhenUnconnected=off
  a_x : Outport  Port=4  VectorParamsAs1DForOutWhenUnconnected=off
  a_y : Outport  Port=5  VectorParamsAs1DForOutWhenUnconnected=off
  a_z : Outport  Port=6  VectorParamsAs1DForOutWhenUnconnected=off
  p : Outport  Port=7  VectorParamsAs1DForOutWhenUnconnected=off
  q : Outport  Port=8  VectorParamsAs1DForOutWhenUnconnected=off
  r : Outport  Port=9  VectorParamsAs1DForOutWhenUnconnected=off
  wires:
  w3/1 -> Attitude Dynamic Model/6(w3)
  w1/1 -> Attitude Dynamic Model/4(w1)
  tau_x/1 -> Attitude Dynamic Model/1(tau_x)
  w2/1 -> Attitude Dynamic Model/5(w2)
  Attitude Dynamic Model/1(p) -> p/1
  w4/1 -> Attitude Dynamic Model/7(w4)
  Attitude Dynamic Model/2(q) -> q/1
  tau_y/1 -> Attitude Dynamic Model/2(tau_y)
  tau_z/1 -> Attitude Dynamic Model/3(tau_z)
  Attitude Dynamic Model/3(r) -> r/1
  qw/1 -> Position Dynamic Model1/1(qw)
  qx/1 -> Position Dynamic Model1/2(qx)
  qy/1 -> Position Dynamic Model1/3(qy)
  qz/1 -> Position Dynamic Model1/4(qz)
  f/1 -> Position Dynamic Model1/5(f)
  Position Dynamic Model1/1(v_x) -> v_x/1
  Position Dynamic Model1/2(v_y) -> v_y/1
  Position Dynamic Model1/3(v_z) -> v_z/1
  Position Dynamic Model1/4(a_x) -> a_x/1
  Position Dynamic Model1/5(a_y) -> a_y/1
  Position Dynamic Model1/6(a_z) -> a_z/1

== system test_without_actuator/混合无人机模型/Quadcopter Dynamics Model/Rigid-Body Kinematic Model ==
  v_x : Inport
  v_y : Inport  Port=2
  v_z : Inport  Port=3
  p : Inport  Port=4
  q : Inport  Port=5
  r : Inport  Port=6
  Attitude Kinematic Model1 : Subsystem
  Position Kinematic Model : Subsystem
  x : Outport  VectorParamsAs1DForOutWhenUnconnected=off
  y : Outport  Port=2  VectorParamsAs1DForOutWhenUnconnected=off
  z : Outport  Port=3  VectorParamsAs1DForOutWhenUnconnected=off
  qw : Outport  Port=4  VectorParamsAs1DForOutWhenUnconnected=off
  qx : Outport  Port=5  VectorParamsAs1DForOutWhenUnconnected=off
  qy : Outport  Port=6  VectorParamsAs1DForOutWhenUnconnected=off
  qz : Outport  Port=7  VectorParamsAs1DForOutWhenUnconnected=off
  wires:
  v_x/1 -> Position Kinematic Model/1(v_x)
  v_y/1 -> Position Kinematic Model/2(v_y)
  r/1 -> Attitude Kinematic Model1/3(r)
  p/1 -> Attitude Kinematic Model1/1(p)
  v_z/1 -> Position Kinematic Model/3(v_z)
  Position Kinematic Model/1(x) -> x/1
  Position Kinematic Model/2(y) -> y/1
  q/1 -> Attitude Kinematic Model1/2(q)
  Position Kinematic Model/3(z) -> z/1
  Attitude Kinematic Model1/2(qx) -> qx/1
  Attitude Kinematic Model1/1(qw) -> qw/1
  Attitude Kinematic Model1/3(qy) -> qy/1
  Attitude Kinematic Model1/4(qz) -> qz/1

== system test_without_actuator/混合无人机模型1/Quadcopter Dynamics Model/Control Effectiveness Model ==
  w1 : Inport
  w2 : Inport  Port=2
  w3 : Inport  Port=3
  w4 : Inport  Port=4
  p : Inport  Port=5
  Eta : Inport  Port=6
  Constant : Constant  Value=ModelParam_c_T
  Constant1 : Constant  Value=ModelParam_c_M
  Constant2 : Constant  Value=ModelParam_d
  MATLAB Function : MATLAB Function  TreatAsAtomicUnit=on  SystemSampleTime=0.1
  f : Outport  VectorParamsAs1DForOutWhenUnconnected=off
  tau_x : Outport  Port=2  VectorParamsAs1DForOutWhenUnconnected=off
  tau_y : Outport  Port=3  VectorParamsAs1DForOutWhenUnconnected=off
  tau_z : Outport  Port=4  VectorParamsAs1DForOutWhenUnconnected=off
  wires:
  Constant1/1 -> MATLAB Function/6(c_M)
  Constant/1 -> MATLAB Function/5(c_T)
  MATLAB Function/3(tau_y) -> tau_y/1
  MATLAB Function/1(f) -> f/1
  Constant2/1 -> MATLAB Function/7(d)
  MATLAB Function/4(tau_z) -> tau_z/1
  w3/1 -> MATLAB Function/3(w3)
  w1/1 -> MATLAB Function/1(w1)
  w4/1 -> MATLAB Function/4(w4)
  MATLAB Function/2(tau_x) -> tau_x/1
  w2/1 -> MATLAB Function/2(w2)
  p/1 -> MATLAB Function/8(p)
  Eta/1 -> MATLAB Function/9(Eta)

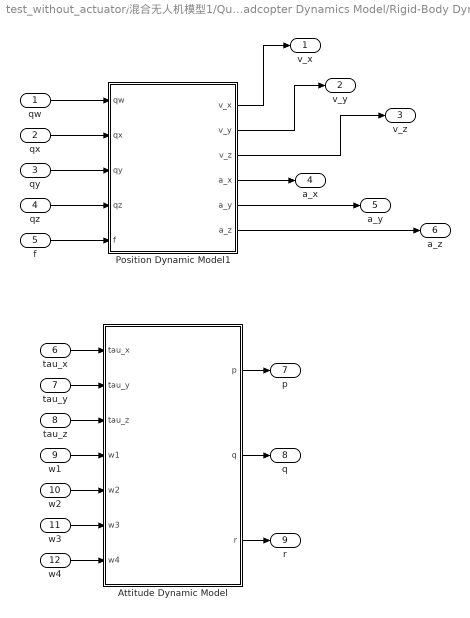
== system test_without_actuator/混合无人机模型1/Quadcopter Dynamics Model/Rigid-Body Dynamic Model ==
  qw : Inport
  qx : Inport  Port=2
  qy : Inport  Port=3
  qz : Inport  Port=4
  f : Inport  Port=5
  tau_x : Inport  Port=6
  tau_y : Inport  Port=7
  tau_z : Inport  Port=8
  w1 : Inport  Port=9
  w2 : Inport  Port=10
  w3 : Inport  Port=11
  w4 : Inport  Port=12
  Attitude Dynamic Model : Subsystem
  Position Dynamic Model1 : Subsystem
  v_x : Outport  VectorParamsAs1DForOutWhenUnconnected=off
  v_y : Outport  Port=2  VectorParamsAs1DForOutWhenUnconnected=off
  v_z : Outport  Port=3  VectorParamsAs1DForOutWhenUnconnected=off
  a_x : Outport  Port=4  VectorParamsAs1DForOutWhenUnconnected=off
  a_y : Outport  Port=5  VectorParamsAs1DForOutWhenUnconnected=off
  a_z : Outport  Port=6  VectorParamsAs1DForOutWhenUnconnected=off
  p : Outport  Port=7  VectorParamsAs1DForOutWhenUnconnected=off
  q : Outport  Port=8  VectorParamsAs1DForOutWhenUnconnected=off
  r : Outport  Port=9  VectorParamsAs1DForOutWhenUnconnected=off
  wires:
  w3/1 -> Attitude Dynamic Model/6(w3)
  w1/1 -> Attitude Dynamic Model/4(w1)
  tau_x/1 -> Attitude Dynamic Model/1(tau_x)
  w2/1 -> Attitude Dynamic Model/5(w2)
  Attitude Dynamic Model/1(p) -> p/1
  w4/1 -> Attitude Dynamic Model/7(w4)
  Attitude Dynamic Model/2(q) -> q/1
  tau_y/1 -> Attitude Dynamic Model/2(tau_y)
  tau_z/1 -> Attitude Dynamic Model/3(tau_z)
  Attitude Dynamic Model/3(r) -> r/1
  qw/1 -> Position Dynamic Model1/1(qw)
  qx/1 -> Position Dynamic Model1/2(qx)
  qy/1 -> Position Dynamic Model1/3(qy)
  qz/1 -> Position Dynamic Model1/4(qz)
  f/1 -> Position Dynamic Model1/5(f)
  Position Dynamic Model1/1(v_x) -> v_x/1
  Position Dynamic Model1/2(v_y) -> v_y/1
  Position Dynamic Model1/3(v_z) -> v_z/1
  Position Dynamic Model1/4(a_x) -> a_x/1
  Position Dynamic Model1/5(a_y) -> a_y/1
  Position Dynamic Model1/6(a_z) -> a_z/1

== system test_without_actuator/混合无人机模型1/Quadcopter Dynamics Model/Rigid-Body Kinematic Model ==
  v_x : Inport
  v_y : Inport  Port=2
  v_z : Inport  Port=3
  p : Inport  Port=4
  q : Inport  Port=5
  r : Inport  Port=6
  Attitude Kinematic Model1 : Subsystem
  Position Kinematic Model : Subsystem
  x : Outport  VectorParamsAs1DForOutWhenUnconnected=off
  y : Outport  Port=2  VectorParamsAs1DForOutWhenUnconnected=off
  z : Outport  Port=3  VectorParamsAs1DForOutWhenUnconnected=off
  qw : Outport  Port=4  VectorParamsAs1DForOutWhenUnconnected=off
  qx : Outport  Port=5  VectorParamsAs1DForOutWhenUnconnected=off
  qy : Outport  Port=6  VectorParamsAs1DForOutWhenUnconnected=off
  qz : Outport  Port=7  VectorParamsAs1DForOutWhenUnconnected=off
  wires:
  v_x/1 -> Position Kinematic Model/1(v_x)
  v_y/1 -> Position Kinematic Model/2(v_y)
  r/1 -> Attitude Kinematic Model1/3(r)
  p/1 -> Attitude Kinematic Model1/1(p)
  v_z/1 -> Position Kinematic Model/3(v_z)
  Position Kinematic Model/1(x) -> x/1
  Position Kinematic Model/2(y) -> y/1
  q/1 -> Attitude Kinematic Model1/2(q)
  Position Kinematic Model/3(z) -> z/1
  Attitude Kinematic Model1/2(qx) -> qx/1
  Attitude Kinematic Model1/1(qw) -> qw/1
  Attitude Kinematic Model1/3(qy) -> qy/1
  Attitude Kinematic Model1/4(qz) -> qz/1

== system test_without_actuator/混合无人机模型2/Quadcopter Dynamics Model/Control Effectiveness Model ==
  w1 : Inport
  w2 : Inport  Port=2
  w3 : Inport  Port=3
  w4 : Inport  Port=4
  p : Inport  Port=5
  Eta : Inport  Port=6
  Constant : Constant  Value=ModelParam_c_T
  Constant1 : Constant  Value=ModelParam_c_M
  Constant2 : Constant  Value=ModelParam_d
  MATLAB Function : MATLAB Function  TreatAsAtomicUnit=on  SystemSampleTime=0.1
  f : Outport  VectorParamsAs1DForOutWhenUnconnected=off
  tau_x : Outport  Port=2  VectorParamsAs1DForOutWhenUnconnected=off
  tau_y : Outport  Port=3  VectorParamsAs1DForOutWhenUnconnected=off
  tau_z : Outport  Port=4  VectorParamsAs1DForOutWhenUnconnected=off
  wires:
  Constant1/1 -> MATLAB Function/6(c_M)
  Constant/1 -> MATLAB Function/5(c_T)
  MATLAB Function/3(tau_y) -> tau_y/1
  MATLAB Function/1(f) -> f/1
  Constant2/1 -> MATLAB Function/7(d)
  MATLAB Function/4(tau_z) -> tau_z/1
  w3/1 -> MATLAB Function/3(w3)
  w1/1 -> MATLAB Function/1(w1)
  w4/1 -> MATLAB Function/4(w4)
  MATLAB Function/2(tau_x) -> tau_x/1
  w2/1 -> MATLAB Function/2(w2)
  p/1 -> MATLAB Function/8(p)
  Eta/1 -> MATLAB Function/9(Eta)

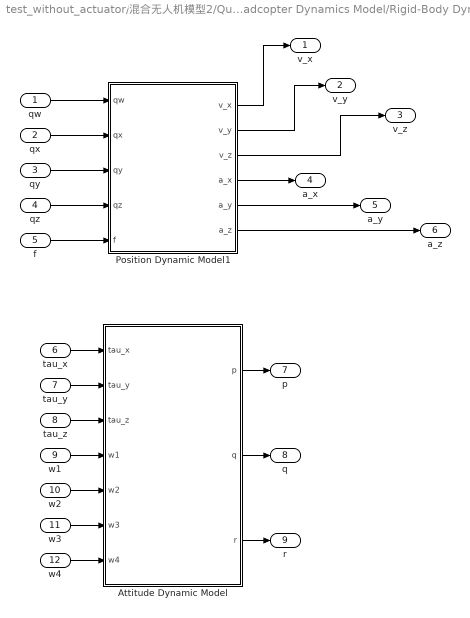
== system test_without_actuator/混合无人机模型2/Quadcopter Dynamics Model/Rigid-Body Dynamic Model ==
  qw : Inport
  qx : Inport  Port=2
  qy : Inport  Port=3
  qz : Inport  Port=4
  f : Inport  Port=5
  tau_x : Inport  Port=6
  tau_y : Inport  Port=7
  tau_z : Inport  Port=8
  w1 : Inport  Port=9
  w2 : Inport  Port=10
  w3 : Inport  Port=11
  w4 : Inport  Port=12
  Attitude Dynamic Model : Subsystem
  Position Dynamic Model1 : Subsystem
  v_x : Outport  VectorParamsAs1DForOutWhenUnconnected=off
  v_y : Outport  Port=2  VectorParamsAs1DForOutWhenUnconnected=off
  v_z : Outport  Port=3  VectorParamsAs1DForOutWhenUnconnected=off
  a_x : Outport  Port=4  VectorParamsAs1DForOutWhenUnconnected=off
  a_y : Outport  Port=5  VectorParamsAs1DForOutWhenUnconnected=off
  a_z : Outport  Port=6  VectorParamsAs1DForOutWhenUnconnected=off
  p : Outport  Port=7  VectorParamsAs1DForOutWhenUnconnected=off
  q : Outport  Port=8  VectorParamsAs1DForOutWhenUnconnected=off
  r : Outport  Port=9  VectorParamsAs1DForOutWhenUnconnected=off
  wires:
  w3/1 -> Attitude Dynamic Model/6(w3)
  w1/1 -> Attitude Dynamic Model/4(w1)
  tau_x/1 -> Attitude Dynamic Model/1(tau_x)
  w2/1 -> Attitude Dynamic Model/5(w2)
  Attitude Dynamic Model/1(p) -> p/1
  w4/1 -> Attitude Dynamic Model/7(w4)
  Attitude Dynamic Model/2(q) -> q/1
  tau_y/1 -> Attitude Dynamic Model/2(tau_y)
  tau_z/1 -> Attitude Dynamic Model/3(tau_z)
  Attitude Dynamic Model/3(r) -> r/1
  qw/1 -> Position Dynamic Model1/1(qw)
  qx/1 -> Position Dynamic Model1/2(qx)
  qy/1 -> Position Dynamic Model1/3(qy)
  qz/1 -> Position Dynamic Model1/4(qz)
  f/1 -> Position Dynamic Model1/5(f)
  Position Dynamic Model1/1(v_x) -> v_x/1
  Position Dynamic Model1/2(v_y) -> v_y/1
  Position Dynamic Model1/3(v_z) -> v_z/1
  Position Dynamic Model1/4(a_x) -> a_x/1
  Position Dynamic Model1/5(a_y) -> a_y/1
  Position Dynamic Model1/6(a_z) -> a_z/1

== system test_without_actuator/混合无人机模型2/Quadcopter Dynamics Model/Rigid-Body Kinematic Model ==
  v_x : Inport
  v_y : Inport  Port=2
  v_z : Inport  Port=3
  p : Inport  Port=4
  q : Inport  Port=5
  r : Inport  Port=6
  Attitude Kinematic Model1 : Subsystem
  Position Kinematic Model : Subsystem
  x : Outport  VectorParamsAs1DForOutWhenUnconnected=off
  y : Outport  Port=2  VectorParamsAs1DForOutWhenUnconnected=off
  z : Outport  Port=3  VectorParamsAs1DForOutWhenUnconnected=off
  qw : Outport  Port=4  VectorParamsAs1DForOutWhenUnconnected=off
  qx : Outport  Port=5  VectorParamsAs1DForOutWhenUnconnected=off
  qy : Outport  Port=6  VectorParamsAs1DForOutWhenUnconnected=off
  qz : Outport  Port=7  VectorParamsAs1DForOutWhenUnconnected=off
  wires:
  v_x/1 -> Position Kinematic Model/1(v_x)
  v_y/1 -> Position Kinematic Model/2(v_y)
  r/1 -> Attitude Kinematic Model1/3(r)
  p/1 -> Attitude Kinematic Model1/1(p)
  v_z/1 -> Position Kinematic Model/3(v_z)
  Position Kinematic Model/1(x) -> x/1
  Position Kinematic Model/2(y) -> y/1
  q/1 -> Attitude Kinematic Model1/2(q)
  Position Kinematic Model/3(z) -> z/1
  Attitude Kinematic Model1/2(qx) -> qx/1
  Attitude Kinematic Model1/1(qw) -> qw/1
  Attitude Kinematic Model1/3(qy) -> qy/1
  Attitude Kinematic Model1/4(qz) -> qz/1

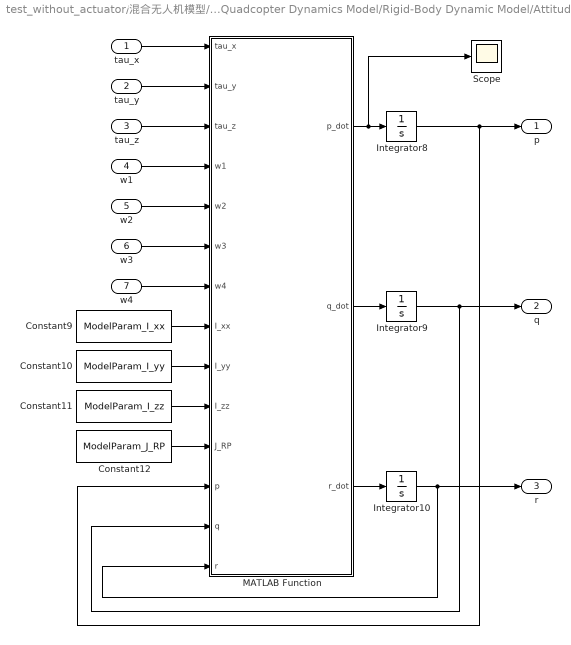
== system test_without_actuator/混合无人机模型/Quadcopter Dynamics Model/Rigid-Body Dynamic Model/Attitude Dynamic Model ==
  tau_x : Inport
  tau_y : Inport  Port=2
  tau_z : Inport  Port=3
  w1 : Inport  Port=4
  w2 : Inport  Port=5
  w3 : Inport  Port=6
  w4 : Inport  Port=7
  Constant10 : Constant  Value=ModelParam_I_yy
  Constant11 : Constant  Value=ModelParam_I_zz
  Constant12 : Constant  Value=ModelParam_J_RP
  Constant9 : Constant  Value=ModelParam_I_xx
  Integrator10 : Integrator
  Integrator8 : Integrator
  Integrator9 : Integrator
  MATLAB Function : MATLAB Function  TreatAsAtomicUnit=on
  Scope : Scope
  p : Outport  VectorParamsAs1DForOutWhenUnconnected=off
  q : Outport  Port=2  VectorParamsAs1DForOutWhenUnconnected=off
  r : Outport  Port=3  VectorParamsAs1DForOutWhenUnconnected=off
  wires:
  Constant9/1 -> MATLAB Function/8(I_xx)
  tau_z/1 -> MATLAB Function/3(tau_z)
  Integrator10/1 -> r/1, MATLAB Function/14(r)
  Constant12/1 -> MATLAB Function/11(J_RP)
  Integrator9/1 -> q/1, MATLAB Function/13(q)
  Constant10/1 -> MATLAB Function/9(I_yy)
  MATLAB Function/3(r_dot) -> Integrator10/1
  MATLAB Function/1(p_dot) -> Scope/1, Integrator8/1
  Integrator8/1 -> p/1, MATLAB Function/12(p)
  tau_y/1 -> MATLAB Function/2(tau_y)
  MATLAB Function/2(q_dot) -> Integrator9/1
  Constant11/1 -> MATLAB Function/10(I_zz)
  w1/1 -> MATLAB Function/4(w1)
  tau_x/1 -> MATLAB Function/1(tau_x)
  w2/1 -> MATLAB Function/5(w2)
  w3/1 -> MATLAB Function/6(w3)
  w4/1 -> MATLAB Function/7(w4)

== system test_without_actuator/混合无人机模型/Quadcopter Dynamics Model/Rigid-Body Dynamic Model/Position Dynamic Model1 ==
  qw : Inport
  qx : Inport  Port=2
  qy : Inport  Port=3
  qz : Inport  Port=4
  f : Inport  Port=5
  Constant7 : Constant  Value=ModelParam_m
  Constant8 : Constant  Value=ModelParam_g
  Integrator1 : Integrator
  Integrator3 : Integrator
  Integrator6 : Integrator
  MATLAB Function : MATLAB Function  TreatAsAtomicUnit=on
  v_x : Outport  VectorParamsAs1DForOutWhenUnconnected=off
  v_y : Outport  Port=2  VectorParamsAs1DForOutWhenUnconnected=off
  v_z : Outport  Port=3  VectorParamsAs1DForOutWhenUnconnected=off
  a_x : Outport  Port=4  VectorParamsAs1DForOutWhenUnconnected=off
  a_y : Outport  Port=5  VectorParamsAs1DForOutWhenUnconnected=off
  a_z : Outport  Port=6  VectorParamsAs1DForOutWhenUnconnected=off
  wires:
  Constant8/1 -> MATLAB Function/2(g)
  MATLAB Function/1(v_x_dot) -> a_x/1, Integrator6/1
  MATLAB Function/2(v_y_dot) -> a_y/1, Integrator1/1
  qx/1 -> MATLAB Function/4(qx)
  Constant7/1 -> MATLAB Function/1(m)
  MATLAB Function/3(v_z_dot) -> a_z/1, Integrator3/1
  qw/1 -> MATLAB Function/3(qw)
  f/1 -> MATLAB Function/7(f)
  qy/1 -> MATLAB Function/5(qy)
  Integrator6/1 -> v_x/1
  Integrator1/1 -> v_y/1
  Integrator3/1 -> v_z/1
  qz/1 -> MATLAB Function/6(qz)

== system test_without_actuator/混合无人机模型/Quadcopter Dynamics Model/Rigid-Body Kinematic Model/Attitude Kinematic Model1 ==
  p : Inport
  q : Inport  Port=2
  r : Inport  Port=3
  Constant1 : Constant  Value=ModelInit_Att_qw
  Constant2 : Constant  Value=ModelInit_Att_qy
  Constant3 : Constant  Value=ModelInit_Att_qz
  Constant4 : Constant  Value=ModelInit_Att_qx
  Integrator{1,3..5} (4 alike) : Integrator  InitialConditionSource=external
  MATLAB Function1 : MATLAB Function  TreatAsAtomicUnit=on
  MATLAB Function2 : MATLAB Function  TreatAsAtomicUnit=on
  qw : Outport  VectorParamsAs1DForOutWhenUnconnected=off
  qx : Outport  Port=2  VectorParamsAs1DForOutWhenUnconnected=off
  qy : Outport  Port=3  VectorParamsAs1DForOutWhenUnconnected=off
  qz : Outport  Port=4  VectorParamsAs1DForOutWhenUnconnected=off
  wires:
  r/1 -> MATLAB Function2/3(r)
  MATLAB Function2/1(qw_dot) -> Integrator3/1
  q/1 -> MATLAB Function2/2(q)
  p/1 -> MATLAB Function2/1(p)
  Constant1/1 -> Integrator3/2
  Constant2/1 -> Integrator4/2
  Constant3/1 -> Integrator5/2
  MATLAB Function2/2(qx_dot) -> Integrator1/1
  Constant4/1 -> Integrator1/2
  MATLAB Function2/3(qy_dot) -> Integrator4/1
  MATLAB Function2/4(qz_dot) -> Integrator5/1
  Integrator3/1 -> MATLAB Function1/1(qw)
  Integrator1/1 -> MATLAB Function1/2(qx)
  Integrator4/1 -> MATLAB Function1/3(qy)
  Integrator5/1 -> MATLAB Function1/4(qz)
  MATLAB Function1/1(qw_unit) -> MATLAB Function2/4(qw), qw/1
  MATLAB Function1/2(qx_unit) -> MATLAB Function2/5(qx), qx/1
  MATLAB Function1/3(qy_unit) -> MATLAB Function2/6(qy), qy/1
  MATLAB Function1/4(qz_unit) -> MATLAB Function2/7(qz), qz/1

== system test_without_actuator/混合无人机模型/Quadcopter Dynamics Model/Rigid-Body Kinematic Model/Position Kinematic Model ==
  v_x : Inport
  v_y : Inport  Port=2
  v_z : Inport  Port=3
  Constant1 : Constant  Value=ModelInit_Pos_z
  Constant2 : Constant  Value=ModelInit_Pos_y
  Constant3 : Constant  Value=ModelInit_Pos_x
  Integrator : Integrator  InitialConditionSource=external
  Integrator1 : Integrator  InitialConditionSource=external
  Integrator2 : Integrator  InitialConditionSource=external
  x : Outport  VectorParamsAs1DForOutWhenUnconnected=off
  y : Outport  Port=2  VectorParamsAs1DForOutWhenUnconnected=off
  z : Outport  Port=3  VectorParamsAs1DForOutWhenUnconnected=off
  wires:
  v_z/1 -> Integrator2/1
  Integrator1/1 -> y/1
  Integrator/1 -> x/1
  Constant1/1 -> Integrator2/2
  Integrator2/1 -> z/1
  v_x/1 -> Integrator/1
  v_y/1 -> Integrator1/1
  Constant2/1 -> Integrator1/2
  Constant3/1 -> Integrator/2

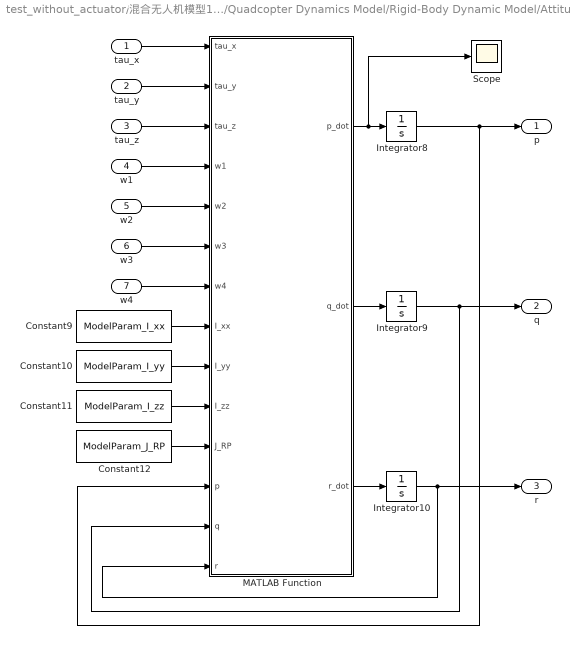
== system test_without_actuator/混合无人机模型1/Quadcopter Dynamics Model/Rigid-Body Dynamic Model/Attitude Dynamic Model ==
  tau_x : Inport
  tau_y : Inport  Port=2
  tau_z : Inport  Port=3
  w1 : Inport  Port=4
  w2 : Inport  Port=5
  w3 : Inport  Port=6
  w4 : Inport  Port=7
  Constant10 : Constant  Value=ModelParam_I_yy
  Constant11 : Constant  Value=ModelParam_I_zz
  Constant12 : Constant  Value=ModelParam_J_RP
  Constant9 : Constant  Value=ModelParam_I_xx
  Integrator10 : Integrator
  Integrator8 : Integrator
  Integrator9 : Integrator
  MATLAB Function : MATLAB Function  TreatAsAtomicUnit=on  SystemSampleTime=0.1
  Scope : Scope
  p : Outport  VectorParamsAs1DForOutWhenUnconnected=off
  q : Outport  Port=2  VectorParamsAs1DForOutWhenUnconnected=off
  r : Outport  Port=3  VectorParamsAs1DForOutWhenUnconnected=off
  wires:
  Constant9/1 -> MATLAB Function/8(I_xx)
  tau_z/1 -> MATLAB Function/3(tau_z)
  Integrator10/1 -> r/1, MATLAB Function/14(r)
  Constant12/1 -> MATLAB Function/11(J_RP)
  Integrator9/1 -> q/1, MATLAB Function/13(q)
  Constant10/1 -> MATLAB Function/9(I_yy)
  MATLAB Function/3(r_dot) -> Integrator10/1
  MATLAB Function/1(p_dot) -> Scope/1, Integrator8/1
  Integrator8/1 -> p/1, MATLAB Function/12(p)
  tau_y/1 -> MATLAB Function/2(tau_y)
  MATLAB Function/2(q_dot) -> Integrator9/1
  Constant11/1 -> MATLAB Function/10(I_zz)
  w1/1 -> MATLAB Function/4(w1)
  tau_x/1 -> MATLAB Function/1(tau_x)
  w2/1 -> MATLAB Function/5(w2)
  w3/1 -> MATLAB Function/6(w3)
  w4/1 -> MATLAB Function/7(w4)

== system test_without_actuator/混合无人机模型1/Quadcopter Dynamics Model/Rigid-Body Dynamic Model/Position Dynamic Model1 ==
  qw : Inport  SampleTime=0.1
  qx : Inport  Port=2
  qy : Inport  Port=3
  qz : Inport  Port=4
  f : Inport  Port=5
  Constant7 : Constant  Value=ModelParam_m  SampleTime=0.1
  Constant8 : Constant  Value=ModelParam_g  SampleTime=0.1
  Integrator1 : Integrator
  Integrator3 : Integrator
  Integrator6 : Integrator
  MATLAB Function : MATLAB Function  TreatAsAtomicUnit=on  SystemSampleTime=0.1
  v_x : Outport  VectorParamsAs1DForOutWhenUnconnected=off
  v_y : Outport  Port=2  VectorParamsAs1DForOutWhenUnconnected=off
  v_z : Outport  Port=3  VectorParamsAs1DForOutWhenUnconnected=off
  a_x : Outport  Port=4  VectorParamsAs1DForOutWhenUnconnected=off
  a_y : Outport  Port=5  VectorParamsAs1DForOutWhenUnconnected=off
  a_z : Outport  Port=6  VectorParamsAs1DForOutWhenUnconnected=off
  wires:
  Constant8/1 -> MATLAB Function/2(g)
  MATLAB Function/1(v_x_dot) -> a_x/1, Integrator6/1
  MATLAB Function/2(v_y_dot) -> a_y/1, Integrator1/1
  qx/1 -> MATLAB Function/4(qx)
  Constant7/1 -> MATLAB Function/1(m)
  MATLAB Function/3(v_z_dot) -> a_z/1, Integrator3/1
  qw/1 -> MATLAB Function/3(qw)
  f/1 -> MATLAB Function/7(f)
  qy/1 -> MATLAB Function/5(qy)
  Integrator6/1 -> v_x/1
  Integrator1/1 -> v_y/1
  Integrator3/1 -> v_z/1
  qz/1 -> MATLAB Function/6(qz)
